simulink model "sampleModel1915"  (R2023a)
settings: Solver=VariableStepAuto  StartTime=0.0  StopTime=10.0  RelTol=1e-3
libraries: hdlsllib x10, simulink x1
settings Model: Creator=user1  LastModifiedBy=user1

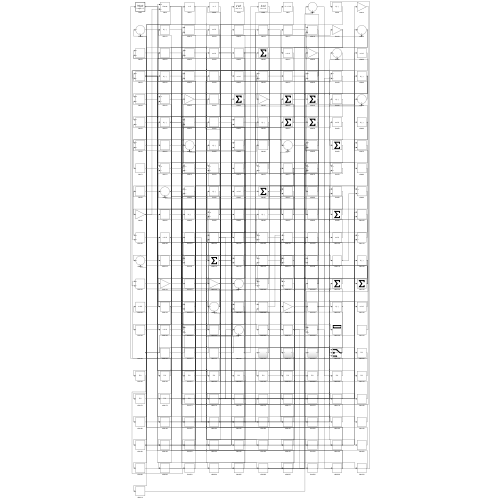
[thumbnail: Simulink's stored preview of the top-level diagram]
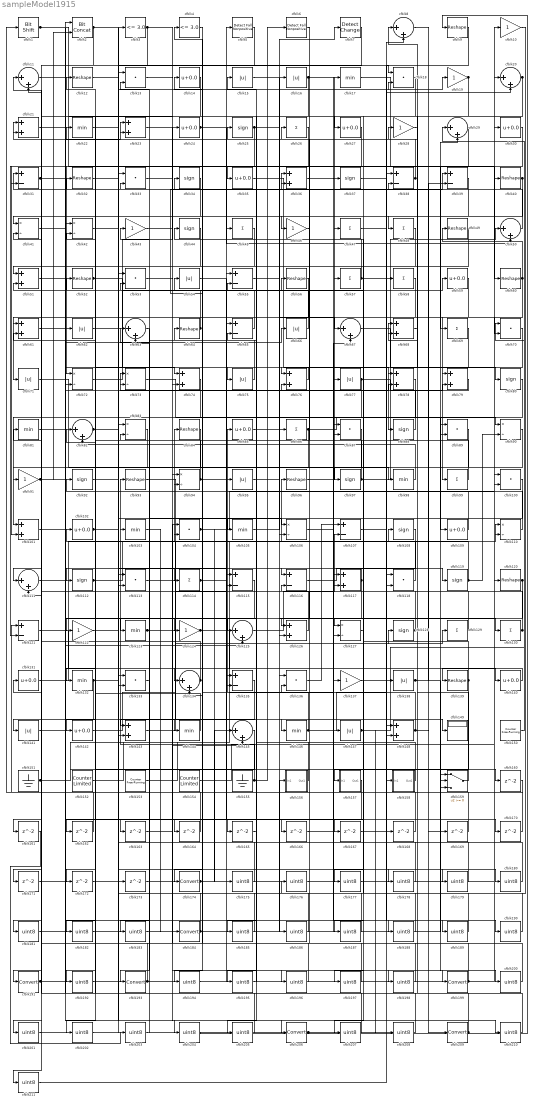
== system sampleModel1915 ==
  cfblk1 : hdlsllib/Logic and Bit Operations/Bit Shift  mode=Shift Left Logical  N=0
  cfblk{10,19,28,43,46,91,122,124,137} (9 alike) : Gain
  cfblk{13,18,33,53,70,87,89,100,104,113,118,133,136} (13 alike) : DotProduct  OutDataTypeStr=Inherit: Inherit via internal rule
  cfblk{21,23,36,51,61,68,74,76,78..79,101,117,126,143,148} (15 alike) : Sum
  cfblk{14,24,27,30,35,59,85,102,109,131,140,142} (12 alike) : Bias  Bias=0.0  SaturateOnIntegerOverflow=off
  cfblk{17,22,81,98,103,105,123,132,144,146} (10 alike) : MinMax
  cfblk{41..42,72..73,83,90,94,106,110,127} (10 alike) : Product  Inputs=*/  RndMeth=Zero  SaturateOnIntegerOverflow=on
  cfblk{31,38..39,55,65,107,115..116,121,135} (10 alike) : Sum  Inputs=+-
  cfblk{25,34,37,44,80,88,92,97,108,112,119,128} (12 alike) : Signum
  cfblk{8,11,20,29,50,63,67,82,111,125,134,145} (12 alike) : Sum  Inputs=|++
  cfblk{26,45,47..48,57..58,69,86,99,114,129..130} (12 alike) : Sum  Inputs=+
  cfblk{9,12,32,40,49,52,56,60,64,84,93,96,120,139} (14 alike) : Reshape
  cfblk{15..16,54,62,66,71,75,77,95,138,141,147} (12 alike) : Abs  SaturateOnIntegerOverflow=off
  cfblk149 : Display
  cfblk150 : hdlsllib/Sources/Counter Free-Running  NumBits=16  tsamp=-1
  cfblk151 : Ground
  cfblk152 : hdlsllib/Sources/Counter Limited  uplimit=7  tsamp=-1
  cfblk153 : hdlsllib/Sources/Counter Free-Running  NumBits=16  tsamp=-1
  cfblk154 : hdlsllib/Sources/Counter Limited  uplimit=7  tsamp=-1
  cfblk155 : Ground
  cfblk156 : Subsystem
      settings: LibrarySourceBlock=|
      | hdlsllib/Ports &
      | Subsystems/Subsystem
  cfblk157 : Subsystem
      settings: LibrarySourceBlock=|
      | hdlsllib/Ports &
      | Subsystems/Subsystem
  cfblk158 : Subsystem
      settings: LibrarySourceBlock=|
      | hdlsllib/Ports &
      | Subsystems/Subsystem
  cfblk159 : Switch  SaturateOnIntegerOverflow=off  InputSameDT=off
  cfblk{160..173} (14 alike) : Delay  SampleTime=1
  cfblk{174,184,191,193,199,206,209} (7 alike) : DataTypeConversion  SaturateOnIntegerOverflow=off  RndMeth=Floor
  cfblk{175..183,185..190,192,194..198,200..205,207..208,210..211} (31 alike) : DataTypeConversion  OutDataTypeStr=uint8  SaturateOnIntegerOverflow=off  RndMeth=Floor
  cfblk2 : hdlsllib/Logic and Bit Operations/Bit Concat  numInputs=2
  cfblk3 : hdlsllib/Logic and Bit Operations/Compare To Constant  relop=<=  const=3.0  OutDataTypeStr=boolean
  cfblk4 : hdlsllib/Logic and Bit Operations/Compare To Constant  relop=<=  const=3.0  OutDataTypeStr=boolean
  cfblk5 : hdlsllib/Logic and Bit Operations/Detect Fall Nonpositive  vinit=0  OutDataTypeStr=boolean
  cfblk6 : hdlsllib/Logic and Bit Operations/Detect Fall Nonpositive  vinit=0  OutDataTypeStr=boolean
  cfblk7 : simulink/Logic and Bit Operations/Detect Change  vinit=0  OutDataTypeStr=boolean
      settings: LibrarySourceBlock=|
      | hdlsllib/Logic and Bit
      | Operations/Detect
      | Change
  wires:
  cfblk76/1 -> cfblk75/1
  cfblk120/1 -> cfblk167/1, cfblk207/1
  cfblk136/1 -> cfblk107/1
  cfblk85/1 -> cfblk86/1
  cfblk38/1 -> cfblk121/2, cfblk12/1
  cfblk130/1 -> cfblk54/1, cfblk11/2, cfblk15/1
  cfblk118/1 -> cfblk102/1
  cfblk94/1 -> cfblk36/1, cfblk21/1, cfblk159/3
  cfblk110/1 -> cfblk92/1
  cfblk93/1 -> cfblk146/1
  cfblk155/1 -> cfblk93/1, cfblk6/1
  cfblk59/1 -> cfblk99/1
  cfblk96/1 -> cfblk17/1
  cfblk103/1 -> cfblk184/1
  cfblk70/1 -> cfblk79/1
  cfblk129/1 -> cfblk34/1
  cfblk142/1 -> cfblk128/1
  cfblk45/1 -> cfblk191/1
  cfblk71/1 -> cfblk137/1
  cfblk126/1 -> cfblk25/1
  cfblk147/1 -> cfblk29/1, cfblk208/1
  cfblk46/1 -> cfblk116/1
  cfblk67/1 -> cfblk80/1
  cfblk30/1 -> cfblk72/1
  cfblk128/1 -> cfblk127/1, cfblk95/1
  cfblk82/1 -> cfblk32/1, cfblk160/1
  cfblk97/1 -> cfblk50/1, cfblk61/2
  cfblk21/1 -> cfblk138/1
  cfblk131/1 -> cfblk84/1
  cfblk63/1 -> cfblk143/1
  cfblk105/1 -> cfblk16/1
  cfblk144/1 -> cfblk82/1
  cfblk40/1 -> cfblk72/2, cfblk87/2, cfblk187/1
  cfblk148/1 -> cfblk85/1, cfblk169/1
  cfblk80/1 -> cfblk101/1
  cfblk143/1 -> cfblk110/1
  cfblk19/1 -> cfblk76/1, cfblk41/1
  cfblk117/1 -> cfblk112/1, cfblk126/2
  cfblk116/1 -> cfblk119/1
  cfblk125/1 -> cfblk107/2
  cfblk20/1 -> cfblk48/1, cfblk157/1(In1)
  cfblk153/1 -> cfblk108/1
  cfblk73/1 -> cfblk109/1
  cfblk60/1 -> cfblk49/1, cfblk105/1, cfblk70/2
  cfblk123/1 -> cfblk115/1, cfblk210/1
  cfblk154/1 -> cfblk100/2
  cfblk152/1 -> cfblk129/1
  cfblk17/1 -> cfblk60/1
  cfblk146/1 -> cfblk58/1, cfblk23/2
  cfblk72/1 -> cfblk59/1
  cfblk35/1 -> cfblk88/1
  cfblk138/1 -> cfblk39/2, cfblk200/1
  cfblk43/1 -> cfblk199/1
  cfblk132/1 -> cfblk19/1, cfblk211/1
  cfblk56/1 -> cfblk71/1
  cfblk11/1 -> cfblk69/1
  cfblk124/1 -> cfblk140/1, cfblk57/1
  cfblk52/1 -> cfblk74/1, cfblk164/1
  cfblk44/1 -> cfblk142/1
  cfblk122/1 -> cfblk3/1
  cfblk135/1 -> cfblk193/1
  cfblk112/1 -> cfblk96/1, cfblk148/2
  cfblk108/1 -> cfblk133/2
  cfblk62/1 -> cfblk24/1
  cfblk107/1 -> cfblk149/1
  cfblk57/1 -> cfblk20/2, cfblk14/1
  cfblk104/1 -> cfblk30/1, cfblk175/1
  cfblk14/1 -> cfblk132/1
  cfblk156/1(Out1) -> cfblk44/1
  cfblk37/1 -> cfblk148/1
  cfblk16/1 -> cfblk37/1, cfblk125/1
  cfblk75/1 -> cfblk31/1
  cfblk158/1(Out1) -> cfblk73/1
  cfblk113/1 -> cfblk5/1
  cfblk64/1 -> cfblk62/1, cfblk41/2
  cfblk65/1 -> cfblk22/1
  cfblk99/1 -> cfblk36/2
  cfblk139/1 -> cfblk117/1, cfblk197/1
  cfblk141/1 -> cfblk66/1
  cfblk18/1 -> cfblk27/1
  cfblk121/1 -> cfblk147/1
  cfblk28/1 -> cfblk78/1
  cfblk119/1 -> cfblk65/2, cfblk90/2
  cfblk92/1 -> cfblk106/1
  cfblk61/1 -> cfblk130/1
  cfblk111/1 -> cfblk76/2
  cfblk49/1 -> cfblk51/1
  cfblk29/1 -> cfblk124/1
  cfblk98/1 -> cfblk82/2
  cfblk23/1 -> cfblk106/2
  cfblk101/1 -> cfblk134/1
  cfblk88/1 -> cfblk26/1
  cfblk68/1 -> cfblk38/2
  cfblk5/1 -> cfblk134/2
  cfblk86/1 -> cfblk143/2, cfblk90/1
  cfblk36/1 -> cfblk98/1
  cfblk8/1 -> cfblk209/1
  cfblk91/1 -> cfblk23/1, cfblk2/2
  cfblk24/1 -> cfblk50/2, cfblk18/2
  cfblk6/1 -> cfblk46/1
  cfblk41/1 -> cfblk2/1
  cfblk42/1 -> cfblk206/1
  cfblk4/1 -> cfblk174/1
  cfblk100/1 -> cfblk123/1
  cfblk1/1 -> cfblk94/1, cfblk188/1
  cfblk79/1 -> cfblk73/2
  cfblk140/1 -> cfblk139/1
  cfblk150/1 -> cfblk70/1
  cfblk25/1 -> cfblk97/1, cfblk7/1, cfblk101/2
  cfblk39/1 -> cfblk61/1
  cfblk26/1 -> cfblk31/2
  cfblk133/1 -> cfblk63/1
  cfblk95/1 -> cfblk136/1
  cfblk109/1 -> cfblk28/1
  cfblk102/1 -> cfblk122/1, cfblk110/2
  cfblk27/1 -> cfblk35/1
  cfblk53/1 -> cfblk115/2
  cfblk159/1 -> cfblk68/1
  cfblk15/1 -> cfblk67/1
  cfblk151/1 -> cfblk67/2, cfblk159/2
  cfblk134/1 -> cfblk52/1, cfblk51/2
  cfblk2/1 -> cfblk113/2, cfblk18/1, cfblk141/1
  cfblk77/1 -> cfblk79/2, cfblk126/1, cfblk117/2
  cfblk50/1 -> cfblk11/1
  cfblk9/1 -> cfblk118/2
  cfblk12/1 -> cfblk114/1
  cfblk66/1 -> cfblk56/1
  cfblk31/1 -> cfblk144/1, cfblk74/2, cfblk125/2, cfblk166/1
  cfblk114/1 -> cfblk39/1, cfblk78/2
  cfblk7/1 -> cfblk91/1
  cfblk3/1 -> cfblk145/2, cfblk161/1
  cfblk34/1 -> cfblk111/1
  cfblk160/1 -> cfblk1/1
  cfblk115/1 -> cfblk162/1
  cfblk162/1 -> cfblk121/1
  cfblk74/1 -> cfblk163/1
  cfblk164/1 -> cfblk21/2
  cfblk51/1 -> cfblk165/1
  cfblk166/1 -> cfblk87/1
  cfblk167/1 -> cfblk38/1
  cfblk168/1 -> cfblk104/2
  cfblk169/1 -> cfblk94/2
  cfblk54/1 -> cfblk170/1
  cfblk170/1 -> cfblk68/2
  cfblk48/1 -> cfblk171/1
  cfblk171/1 -> cfblk29/2
  cfblk157/1(Out1) -> cfblk172/1
  cfblk172/1 -> cfblk20/1
  cfblk22/1 -> cfblk173/1
  cfblk173/1 -> cfblk65/1
  cfblk174/1 -> cfblk77/1, cfblk145/1, cfblk159/1
  cfblk175/1 -> cfblk4/1
  cfblk10/1 -> cfblk176/1
  cfblk176/1 -> cfblk100/1
  cfblk127/1 -> cfblk177/1
  cfblk177/1 -> cfblk10/1
  cfblk13/1 -> cfblk178/1
  cfblk178/1 -> cfblk136/2
  cfblk32/1 -> cfblk179/1
  cfblk179/1 -> cfblk13/1
  cfblk137/1 -> cfblk180/1
  cfblk180/1 -> cfblk13/2
  cfblk89/1 -> cfblk181/1
  cfblk181/1 -> cfblk156/1(In1)
  cfblk84/1 -> cfblk182/1
  cfblk182/1 -> cfblk89/1
  cfblk78/1 -> cfblk183/1
  cfblk183/1 -> cfblk89/2
  cfblk184/1 -> cfblk127/2, cfblk133/1
  cfblk90/1 -> cfblk185/1
  cfblk185/1 -> cfblk103/1
  cfblk55/1 -> cfblk186/1
  cfblk186/1 -> cfblk53/1
  cfblk187/1 -> cfblk55/1
  cfblk188/1 -> cfblk55/2
  cfblk47/1 -> cfblk189/1
  cfblk189/1 -> cfblk53/2
  cfblk106/1 -> cfblk190/1
  cfblk190/1 -> cfblk47/1
  cfblk191/1 -> cfblk120/1, cfblk40/1
  cfblk145/1 -> cfblk192/1
  cfblk192/1 -> cfblk45/1
  cfblk193/1 -> cfblk111/2, cfblk131/1
  cfblk87/1 -> cfblk194/1
  cfblk194/1 -> cfblk135/1
  cfblk165/1 -> cfblk195/1
  cfblk195/1 -> cfblk135/2
  cfblk33/1 -> cfblk196/1
  cfblk196/1 -> cfblk64/1
  cfblk197/1 -> cfblk33/1
  cfblk163/1 -> cfblk198/1
  cfblk198/1 -> cfblk33/2
  cfblk199/1 -> cfblk116/2, cfblk104/1
  cfblk200/1 -> cfblk43/1
  cfblk83/1 -> cfblk201/1
  cfblk201/1 -> cfblk118/1
  cfblk69/1 -> cfblk202/1
  cfblk202/1 -> cfblk83/1
  cfblk161/1 -> cfblk203/1
  cfblk203/1 -> cfblk83/2
  cfblk81/1 -> cfblk204/1
  cfblk204/1 -> cfblk9/1
  cfblk58/1 -> cfblk205/1
  cfblk205/1 -> cfblk81/1
  cfblk206/1 -> cfblk168/1, cfblk158/1(In1)
  cfblk207/1 -> cfblk42/1
  cfblk208/1 -> cfblk42/2
  cfblk209/1 -> cfblk63/2, cfblk113/1
  cfblk210/1 -> cfblk8/1
  cfblk211/1 -> cfblk8/2

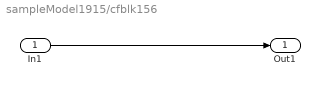
== system sampleModel1915/cfblk156 ==
  In1 : Inport
  Out1 : Outport
  wires:
  In1/1 -> Out1/1

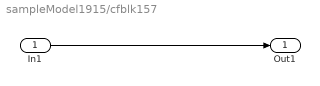
== system sampleModel1915/cfblk157 ==
  In1 : Inport
  Out1 : Outport
  wires:
  In1/1 -> Out1/1

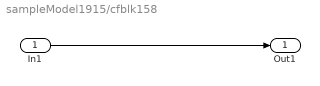
== system sampleModel1915/cfblk158 ==
  In1 : Inport
  Out1 : Outport
  wires:
  In1/1 -> Out1/1
